simulink model "motor_current_speed"  (R2021a)
settings: Solver=VariableStepAuto  StartTime=0.0  StopTime=10  RelTol=1e-3
values from neighbouring files (symbols this model uses):
  J = 1.3*10^-5    (= 1.3e-05)    [Task1.m]    (also in Task2.m = 0.0353077; Task3.m = 0.0353077; Task4.m = y(j,3); Task5.m = param_matrix(i,3))
  K = 0.397    [Task1.m]    (also in Task2.m; Task3.m; Task4.m = y(j,4); Task5.m = param_matrix(i,1))
  L = 0.2*10^-4    (= 2e-05)    [Task1.m]    (also in Task2.m; Task3.m; Task4.m = y(j,2); Task5.m = param_matrix(i,2))
  R = 1.77    [Task1.m]    (also in Task2.m; Task3.m; Task4.m = y(j,1); Task5.m = param_matrix(i,4))
  T_f = 0.115    [Task1.m]    (also in Task2.m = 0.119; Task3.m = 0.119; Task4.m = 0.119; Task5.m = param_matrix(i,5))
  T_l = T_l_range(1,i)    [Task1.m]    (also in Task2.m = 0.52; Task2b.m; Task3.m; Task4.m = T_l_range(1,k))
  V = 12    [Task1.m]    (also in Task2.m; Task2b.m; Task3.m; Task4.m = y(j,5))
settings Model: Creator=Usamat980  LastModifiedBy=Usamat980

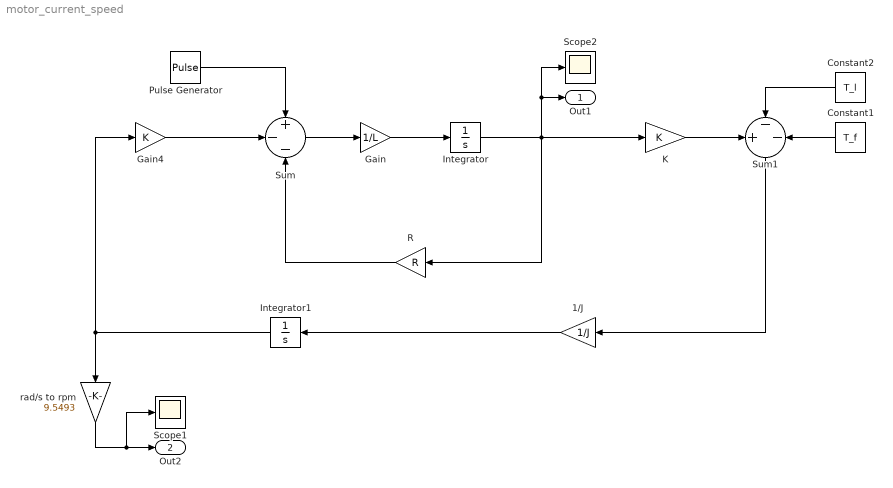
== system motor_current_speed ==
  1/J : Gain  Gain=1/J
  Constant1 : Constant  Value=T_f
  Constant2 : Constant  Value=T_l
  Gain : Gain  Gain=1/L
  Gain4 : Gain  Gain=K
  Integrator : Integrator  LimitOutput=on  UpperSaturationLimit=300  LowerSaturationLimit=0
  Integrator1 : Integrator  LimitOutput=on  UpperSaturationLimit=1000  LowerSaturationLimit=0
  K : Gain  Gain=K
  Pulse Generator : DiscretePulseGenerator  PulseType=Time based  Amplitude=V  Period=20  PulseWidth=99
  R : Gain  Gain=R
  Scope1 : Scope
  Scope2 : Scope
  Sum : Sum  Inputs=+--
  Sum1 : Sum  Inputs=+--
  rad/s to rpm : Gain  Gain=9.5493
  Out1 : Outport
  Out2 : Outport  Port=2
  wires:
  1/J/1 -> Integrator1/1
  Gain/1 -> Integrator/1
  Integrator1/1 -> Gain4/1, rad/s to rpm/1
  R/1 -> Sum/3
  Integrator/1 -> R/1, K/1, Scope2/1, Out1/1
  Sum/1 -> Gain/1
  Pulse Generator/1 -> Sum/1
  rad/s to rpm/1 -> Scope1/1, Out2/1
  Gain4/1 -> Sum/2
  K/1 -> Sum1/1
  Constant2/1 -> Sum1/2
  Constant1/1 -> Sum1/3
  Sum1/1 -> 1/J/1
